simulink model "SimulationModel"  (R2014a)
settings: Solver=ode3  SolverMode=SingleTasking  StartTime=0.0  StopTime=180  FixedStep=deltaT  RelTol=1e-3
PostLoadFcn:
  | loadRobotParameters
  | 
  | allotedRunTime = 3*60; % [sec] Time allowed for run
  | 
  | % starting parameters
  | % The timer starts once the robot has moved a certain distance from the
  | % starting point
  | startPos = [50 50]; % [cm]
  | startingRadius = 10; % [cm]
  | 
  | % Target parameters
  | targetBoundaryRadius = 7; % [cm] radius considered at location
  | statTimeReq = 2.5; % [sec] minimum time robot must be at location
InitFcn:
  | close('all','force');
StartFcn:
  | reset(SimDisplay.getInstance());
undefined symbols (not defined in the file): AxleLength, deltaT, dT, EncL_init, EncR_init, EncRes, motorBiasLeft, motorBiasRight, motorDeadZoneFwd, motorDeadZoneRev, motorGainLeft, motorGainRight, TargetPositions, theta0, Ts, WheelRadius, x0, y0
libraries: simulink x5, opclib x1
CloseFcn:
  | close('all','force');
settings Model: PauseTimes=14  ExtModeTrigDuration=2  Creator=gpacitti  LastModifiedBy=arequet
settings DataIOCC: SignalLoggingSaveFormat=ModelDataLogs  SaveOutput=off  SignalLogging=off  DSMLogging=off  SaveTime=off
settings OptimizationCC: ExpressionDepthLimit=2147483647  OptimizeModelRefInitCode=on  LifeSpan=1
settings DebuggingCC: UnderspecifiedInitializationDetection=Classic  SolverPrmCheckMsg=none  MultiTaskDSMMsg=warning  MultiTaskCondExecSysMsg=none  ParameterPrecisionLossMsg=none  StateNameClashWarn=warning
settings HardwareCC: ProdLargestAtomicInteger=Long  ProdLargestAtomicFloat=Float  ProdEndianess=LittleEndian  ProdHWDeviceType=ARM Compatible->ARM 7
settings RTWCC: SystemTargetFile=ert.tlc  TemplateMakefile=ert_default_tmf  Description=Embedded Coder  RTWVerbose=off  ProcessScript=ert_make_rtw_hook  IncludeERTFirstTime=on
settings CodeAppCC: IgnoreCustomStorageClasses=off  CustomSymbolStrType=$N$R$M  InternalIdentifier=Classic
settings ERTTargetCC: ParMdlRefBuildCompliant=on  CompOptLevelCompliant=on  ConcurrentExecutionCompliant=on  ERTFirstTimeCompliant=on  ModelStepFunctionPrototypeControlCompliant=on  CPPClassGenCompliant=on  InlinedParameterPlacement=Hierarchical  ERTCustomFileTemplate=example_file_process.tlc
settings ConfigComp: Description=Design Verifier Custom Configuration Component  DVMaxTestCaseSteps=500  DVTestSuiteOptimization=CombinedObjectives (Nonlinear Extended)

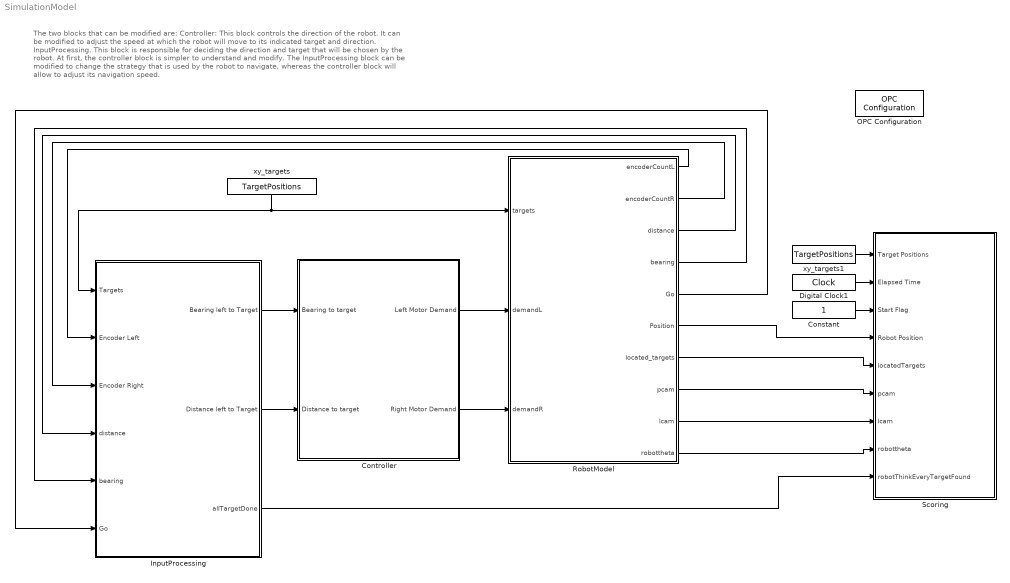
== system SimulationModel ==
  note: The two blocks that can be modified are:
      | Controller: This block controls the direction of the robot. It can be modified to adjust the speed at which the robot will move to its indicated target and direction.
      | InputProcessing. This block is responsible for deciding the direction and target that will be chosen by the robot.
      |
      | At first, the controller block is simpler to understand and modify.
      | The InputProcessing block can be modified to change the strategy that is used by the robot to navigate, whereas the controller block will allow to adjust its navigation speed.
  Constant : Constant  OutDataTypeStr=boolean
  Controller : Subsystem  TreatAsAtomicUnit=on
      mask Display: image('Arduino_Mega_2560.jpg',[0.75/2,0.3,0.25,0.4]);
  Digital Clock1 : DigitalClock  SampleTime=Ts
  InputProcessing : Subsystem
      mask Display: image('Arduino_Mega_2560.jpg',[0.75/2,0.3,0.25,0.3]);
  OPC Configuration : opclib/OPC Configuration  errMissingItems=Error  errReadWrite=Warn  errShutdown=Error  errRTViolation=None  rtEnable=on  speedup=1  showLatency=off  beingUsed=on
  RobotModel : Subsystem
      mask Display: image('robot_3d.jpg',[0.20,0.3,0.45,0.3]);
  Scoring : Subsystem
      mask Display: image('juge.jpg',[0.45,0.3,0.5,0.25]);
  xy_targets : Constant  Value=TargetPositions  OutDataTypeStr=single  SampleTime=1
  xy_targets1 : Constant  Value=TargetPositions  OutDataTypeStr=single  SampleTime=1
  wires:
  RobotModel/2(encoderCountR) -> InputProcessing/3(Encoder Right)
  RobotModel/1(encoderCountL) -> InputProcessing/2(Encoder Left)
  xy_targets/1 -> InputProcessing/1(Targets), RobotModel/1(targets)
  RobotModel/6(Position) -> Scoring/4(Robot Position)
  InputProcessing/2(Distance left to Target) -> Controller/2(Distance to target)
  InputProcessing/1(Bearing left to Target) -> Controller/1(Bearing to target)
  Controller/1(Left Motor Demand) -> RobotModel/2(demandL)
  Controller/2(Right Motor Demand) -> RobotModel/3(demandR)
  Constant/1 -> Scoring/3(Start Flag)
  Digital Clock1/1 -> Scoring/2(Elapsed Time)
  RobotModel/3(distance) -> InputProcessing/4(distance)
  RobotModel/4(bearing) -> InputProcessing/5(bearing)
  RobotModel/7(located_targets) -> Scoring/5(locatedTargets)
  RobotModel/8(pcam) -> Scoring/6(pcam)
  RobotModel/9(lcam) -> Scoring/7(lcam)
  RobotModel/10(robottheta) -> Scoring/8(robottheta)
  InputProcessing/3(allTargetDone) -> Scoring/9(robotThinkEveryTargetFound)
  xy_targets1/1 -> Scoring/1(Target Positions)
  RobotModel/5(Go) -> InputProcessing/6(Go)

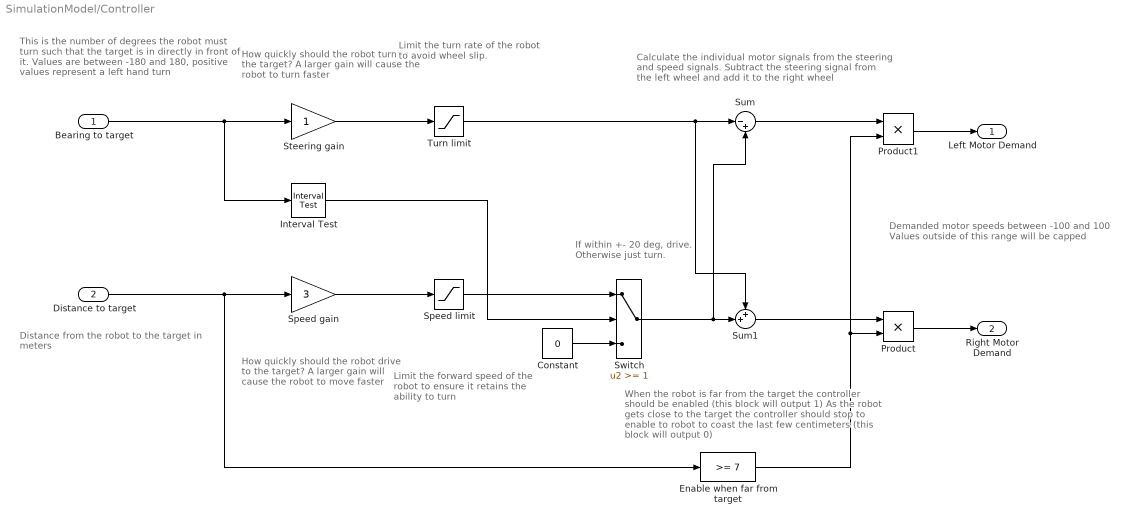
== system SimulationModel/Controller ==
  note: This is the number of degrees the robot
      | must turn such that the target is in directly
      | in front of it.
      | Values are between -180 and 180,
      | positive values represent a left hand turn
  note: Distance from the robot to the target
      | in meters
  note: Demanded motor speeds between -100 and 100
      | Values outside of this range will be capped
  note: How quickly should the robot turn
      | to the target? A larger gain will
      |  cause the robot to turn faster
  note: How quickly should the robot
      | drive to the target? A larger gain
      | will cause the robot to move
      | faster
  note: Limit the forward speed of the
      | robot to ensure it retains the
      | ability to turn
  note: When the robot is far from the target the controller
      | should be enabled (this block will output 1)
      | As the robot gets close to the target the controller
      | should stop to enable to robot to coast the last
      | few centimeters (this block will output 0)
  note: Calculate the individual motor signals from the
      | steering and speed signals. Subtract the steering
      | signal from the left wheel and add it to the right
      | wheel
  note: If within +- 20 deg, drive.
      | Otherwise just turn.
  note: Limit the turn rate of the
      | robot to avoid wheel slip.
  Bearing to target : Inport  OutDataTypeStr=single
  Distance to target : Inport  Port=2  PortDimensions=1  SampleTime=dT
  Constant : Constant  Value=0  OutDataTypeStr=single
  Enable when far from target : simulink/Logic and Bit Operations/Compare To Constant  relop=>=  const=7  OutDataTypeStr=uint8
  Interval Test : simulink/Logic and Bit Operations/Interval Test  IntervalClosedRight=on  uplimit=20  IntervalClosedLeft=on  lowlimit=-20  OutDataTypeStr=boolean
      settings: AttributesFormatString=|
      | Upper = %<uplimit>
      | Lower = %<lowlimit>
  Product : Product
  Product1 : Product
  Speed gain : Gain  Gain=3
  Speed limit : Saturate  UpperLimit=50  LowerLimit=0
      settings: AttributesFormatString=|
      | Upper = %<UpperLimit>
      | Lower = %<LowerLimit>
  Steering gain : Gain
  Sum : Sum  Inputs=|-+
  Sum1 : Sum  Inputs=++|
  Switch : Switch  Threshold=1
  Turn limit : Saturate  UpperLimit=50  LowerLimit=-50
      settings: AttributesFormatString=|
      | Upper = %<UpperLimit>
      | Lower = %<LowerLimit>
  Left Motor Demand : Outport  OutDataTypeStr=single
  Right Motor Demand : Outport  Port=2  OutDataTypeStr=single
  wires:
  Speed limit/1 -> Switch/1
  Turn limit/1 -> Sum1/1, Sum/1
  Constant/1 -> Switch/3
  Interval Test/1 -> Switch/2
  Sum/1 -> Product1/1
  Sum1/1 -> Product/1
  Bearing to target/1 -> Steering gain/1, Interval Test/1
  Switch/1 -> Sum1/2, Sum/2
  Enable when far from target/1 -> Product1/2, Product/2
  Product1/1 -> Left Motor Demand/1
  Product/1 -> Right Motor Demand/1
  Speed gain/1 -> Speed limit/1
  Steering gain/1 -> Turn limit/1
  Distance to target/1 -> Enable when far from target/1, Speed gain/1

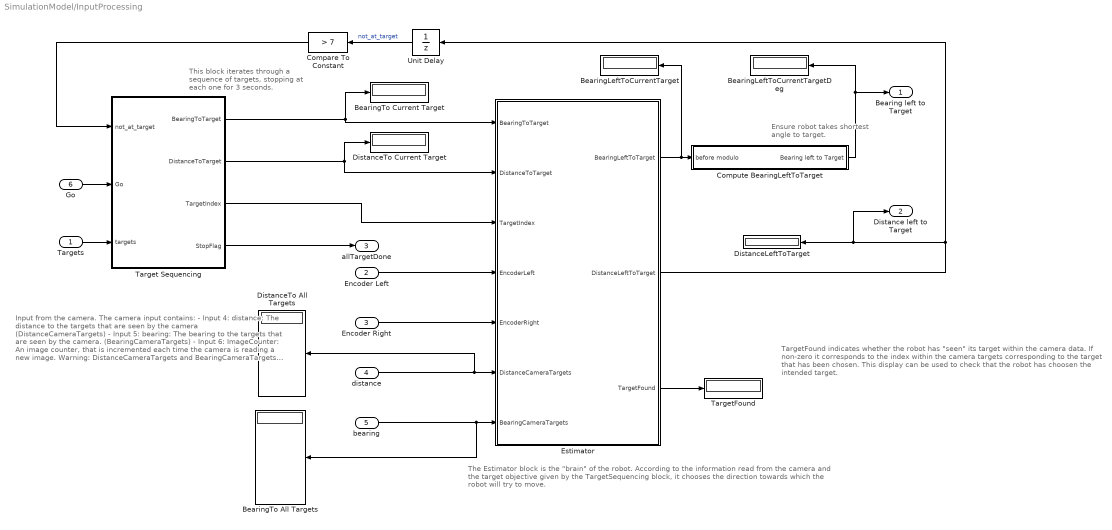
== system SimulationModel/InputProcessing ==
  note: TargetFound indicates whether the robot has "seen" its target within the camera
      | data.
      | If non-zero it corresponds to the index within the camera targets corresponding
      | to the target that has been chosen.
      |
      | This display can be used to check that the robot has choosen the intended
      | target.
  note: The Estimator block is the "brain" of the robot. According to the information read from the camera and the
      | target objective given by the TargetSequencing block, it chooses the direction towards which the robot
      | will try to move.
  note: Ensure robot takes shortest
      | angle to target.
  note: This block iterates through a
      | sequence of targets, stopping
      | at each one for 3 seconds.
  note: Input from the camera. The camera input contains:
      | - Input 4: distance: The distance to the targets that are seen by the
      |   camera (DistanceCameraTargets)
      | - Input 5: bearing: The bearing to the targets that are seen
      |   by the camera. (BearingCameraTargets)
      | - Input 6: ImageCounter: An image counter, that is incremented
      |   each time the camera is reading a new image.
      | Warning: DistanceCameraTargets and BearingCameraTargets
      | are the targets seen by the camera. So for instance, the
      | target 1 is the first target seen by the camera, but is not the
      | same target as the target at index 1 within the target sequencing
      | block.
  Targets : Inport
  Encoder Left : Inport  Port=2  OutDataTypeStr=class(intEncoder(0))
  Encoder Right : Inport  Port=3  OutDataTypeStr=class(intEncoder(0))
  distance : Inport  Port=4
  bearing : Inport  Port=5
  Go : Inport  Port=6
  BearingLeftToCurrentTarget : Display
  BearingLeftToCurrentTargetDeg : Display
  BearingTo All Targets : Display
  "BearingTo Current Target " : Display
  Compare To Constant : simulink/Logic and Bit Operations/Compare To Constant  relop=>  const=7  OutDataTypeStr=boolean
  Compute BearingLeftToTarget : Subsystem
  DistanceLeftToTarget : Display
  DistanceTo All Targets : Display
  DistanceTo Current Target : Display
  Estimator : MATLAB Function  TreatAsAtomicUnit=on
  Target Sequencing : Stateflow chart  TreatAsAtomicUnit=on
  TargetFound : Display
  Unit Delay : UnitDelay  SampleTime=dT
  Bearing left to Target : Outport  SampleTime=dT
  Distance left to Target : Outport  Port=2
  allTargetDone : Outport  Port=3
  wires:
  Go/1 -> Target Sequencing/2(Go)
  distance/1 -> DistanceTo All Targets/1, Estimator/6(DistanceCameraTargets)
  bearing/1 -> Estimator/7(BearingCameraTargets), BearingTo All Targets/1
  Target Sequencing/4(StopFlag) -> allTargetDone/1
  Compare To Constant/1 -> Target Sequencing/1(not_at_target)
  Compute BearingLeftToTarget/1(Bearing left to Target) -> BearingLeftToCurrentTargetDeg/1, Bearing left to Target/1
  Estimator/3(TargetFound) -> TargetFound/1
  Target Sequencing/3(TargetIndex) -> Estimator/3(TargetIndex)
  Estimator/2(DistanceLeftToTarget) -> DistanceLeftToTarget/1, Distance left to Target/1, Unit Delay/1
  Estimator/1(BearingLeftToTarget) -> BearingLeftToCurrentTarget/1, Compute BearingLeftToTarget/1(before modulo)
  Target Sequencing/1(BearingToTarget) -> Estimator/1(BearingToTarget), "BearingTo Current Target "/1
  Unit Delay/1 -> Compare To Constant/1  "not_at_target"
  Encoder Right/1 -> Estimator/5(EncoderRight)
  Target Sequencing/2(DistanceToTarget) -> Estimator/2(DistanceToTarget), DistanceTo Current Target/1
  Encoder Left/1 -> Estimator/4(EncoderLeft)
  Targets/1 -> Target Sequencing/3(targets)

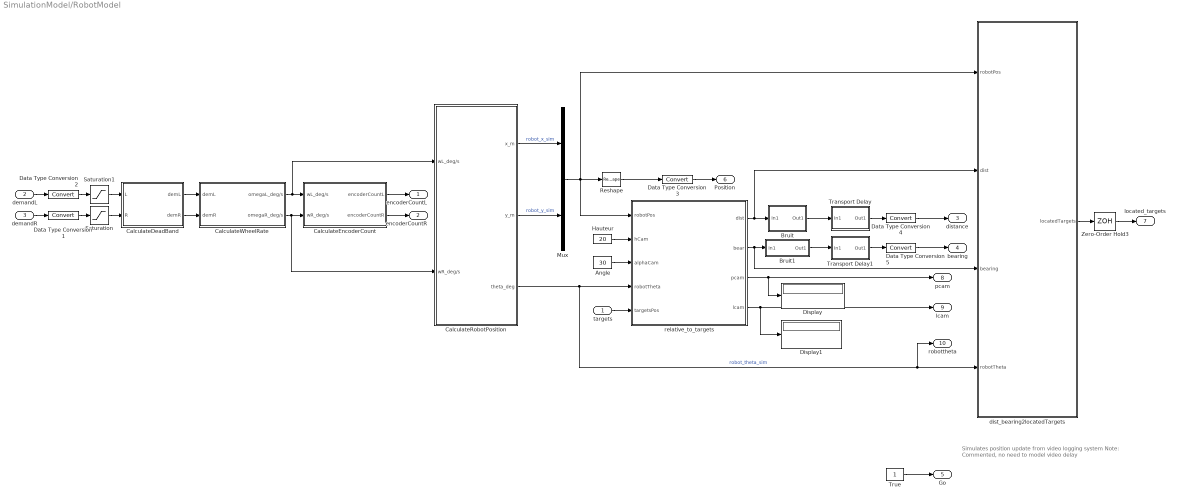
== system SimulationModel/RobotModel ==
  note: Simulates position update from video logging system
      | Note: Commented, no need to model video delay
  targets : Inport
  demandL : Inport  Port=2  SampleTime=0
  demandR : Inport  Port=3  SampleTime=0
  Angle : Constant  Value=30  OutMin=[30]  OutMax=[60]  SampleTime=0.2
  Bruit : Subsystem
  Bruit1 : Subsystem
  CalculateDeadBand : MATLAB Function  TreatAsAtomicUnit=on
  CalculateEncoderCount : Subsystem
  CalculateRobotPosition : Subsystem
  CalculateWheelRate : Subsystem
  Data Type Conversion{1..5} (5 alike) : DataTypeConversion
  Display : Display
  Display1 : Display
  Hauteur : Constant  Value=20  SampleTime=0.2
  Mux : Mux  Inputs=2
  Reshape : Reshape  OutputDimensionality=Row vector (2-D)
  Saturation : Saturate  UpperLimit=100  LowerLimit=-100
  Saturation1 : Saturate  UpperLimit=100  LowerLimit=-100
  Transport Delay : Subsystem  mask{timeDelay=0.250, initialOutput=zeros(size(6,1),1), initialBufferSize=1024, useFixedBufferSize=off, directFeedthoughOfInputDuringLinearization=off, padeOrder=0}
      mask prompts: initialOutput "Initial output"; initialBufferSize "Initial buffer size"; useFixedBufferSize "Use fixed buffer size"; directFeedthoughOfInputDuringLinearization "Direct feedthough of input during linearization"; padeOrder "Pade order (for linearization):"
  Transport Delay1 : Subsystem  mask{timeDelay=0.250, initialOutput=zeros(size(6,1),1), initialBufferSize=1024, useFixedBufferSize=off, directFeedthoughOfInputDuringLinearization=off, padeOrder=0}
      mask prompts: initialOutput "Initial output"; initialBufferSize "Initial buffer size"; useFixedBufferSize "Use fixed buffer size"; directFeedthoughOfInputDuringLinearization "Direct feedthough of input during linearization"; padeOrder "Pade order (for linearization):"
  True : Constant  OutMin=0  OutMax=1  SampleTime=0.1
  Zero-Order Hold3 : ZeroOrderHold  SampleTime=0.2
  dist_bearing2locatedTargets : MATLAB Function  TreatAsAtomicUnit=on
  relative_to_targets : MATLAB Function  TreatAsAtomicUnit=on
  encoderCountL : Outport  OutDataTypeStr=class(intEncoder(0))
  encoderCountR : Outport  Port=2  OutDataTypeStr=class(intEncoder(0))
  distance : Outport  Port=3  OutDataTypeStr=int16
  bearing : Outport  Port=4  OutDataTypeStr=int8
  Go : Outport  Port=5
  Position : Outport  Port=6
  located_targets : Outport  Port=7
  pcam : Outport  Port=8
  lcam : Outport  Port=9
  robottheta : Outport  Port=10
  wires:
  CalculateRobotPosition/1(x_m) -> Mux/1  "robot_x_sim"
  CalculateRobotPosition/2(y_m) -> Mux/2  "robot_y_sim"
  demandR/1 -> Data Type Conversion1/1
  demandL/1 -> Data Type Conversion2/1
  CalculateDeadBand/1(demL) -> CalculateWheelRate/1(demL)
  CalculateDeadBand/2(demR) -> CalculateWheelRate/2(demR)
  Saturation/1 -> CalculateDeadBand/2(R)
  Saturation1/1 -> CalculateDeadBand/1(L)
  CalculateEncoderCount/1(encoderCountL) -> encoderCountL/1
  CalculateEncoderCount/2(encoderCountR) -> encoderCountR/1
  CalculateRobotPosition/3(theta_deg) -> robottheta/1, dist_bearing2locatedTargets/4(robotTheta), relative_to_targets/4(robotTheta)  "robot_theta_sim"
  CalculateWheelRate/1(omegaL_deg/s) -> CalculateEncoderCount/1(wL_deg/s), CalculateRobotPosition/1(wL_deg/s)
  CalculateWheelRate/2(omegaR_deg/s) -> CalculateEncoderCount/2(wR_deg/s), CalculateRobotPosition/2(wR_deg/s)
  Data Type Conversion2/1 -> Saturation1/1
  Data Type Conversion1/1 -> Saturation/1
  Reshape/1 -> Data Type Conversion3/1
  Data Type Conversion3/1 -> Position/1
  targets/1 -> relative_to_targets/5(targetsPos)
  Zero-Order Hold3/1 -> located_targets/1
  dist_bearing2locatedTargets/1(locatedTargets) -> Zero-Order Hold3/1
  relative_to_targets/1(dist) -> Bruit/1(In1), dist_bearing2locatedTargets/2(dist)
  relative_to_targets/2(bear) -> Bruit1/1(In1), dist_bearing2locatedTargets/3(bearing)
  Transport Delay1/1(Out1) -> Data Type Conversion5/1
  Hauteur/1 -> relative_to_targets/2(hCam)
  Bruit1/1(Out1) -> Transport Delay1/1(In1)
  Angle/1 -> relative_to_targets/3(alphaCam)
  relative_to_targets/3(pcam) -> Display/1, pcam/1
  relative_to_targets/4(lcam) -> Display1/1, lcam/1
  Mux/1 -> dist_bearing2locatedTargets/1(robotPos), Reshape/1, relative_to_targets/1(robotPos)
  Bruit/1(Out1) -> Transport Delay/1(In1)
  Transport Delay/1(Out1) -> Data Type Conversion4/1
  Data Type Conversion4/1 -> distance/1
  Data Type Conversion5/1 -> bearing/1
  True/1 -> Go/1

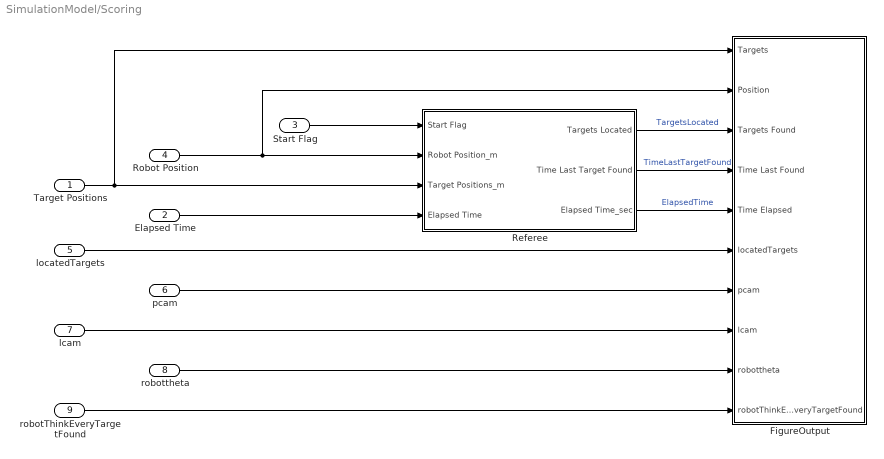
== system SimulationModel/Scoring ==
  Target Positions : Inport
  Elapsed Time : Inport  Port=2
  Start Flag : Inport  Port=3
  Robot Position : Inport  Port=4
  locatedTargets : Inport  Port=5
  pcam : Inport  Port=6
  lcam : Inport  Port=7
  robottheta : Inport  Port=8
  robotThinkEveryTargetFound : Inport  Port=9
  FigureOutput : Subsystem  TreatAsAtomicUnit=on  SimViewingDevice=on
  Referee : Subsystem
      mask Display: % image(imread('referee.png'))
  wires:
  Referee/1(Targets Located) -> FigureOutput/3(Targets Found)  "TargetsLocated"
  Referee/2(Time Last Target Found) -> FigureOutput/4(Time Last Found)  "TimeLastTargetFound"
  Referee/3(Elapsed Time_sec) -> FigureOutput/5(Time Elapsed)  "ElapsedTime"
  Start Flag/1 -> Referee/1(Start Flag)
  Robot Position/1 -> Referee/2(Robot Position_m), FigureOutput/2(Position)
  Elapsed Time/1 -> Referee/4(Elapsed Time)
  Target Positions/1 -> FigureOutput/1(Targets), Referee/3(Target Positions_m)
  locatedTargets/1 -> FigureOutput/6(locatedTargets)
  pcam/1 -> FigureOutput/7(pcam)
  lcam/1 -> FigureOutput/8(lcam)
  robottheta/1 -> FigureOutput/9(robottheta)
  robotThinkEveryTargetFound/1 -> FigureOutput/10(robotThinkEveryTargetFound)

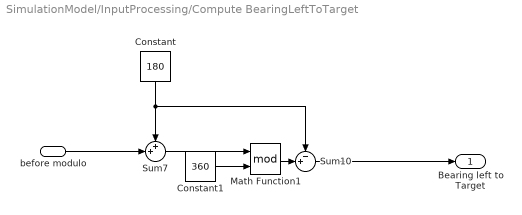
== system SimulationModel/InputProcessing/Compute BearingLeftToTarget ==
  before modulo : Inport
  Constant : Constant  Value=180  OutDataTypeStr=Inherit: Inherit via back propagation
  Constant1 : Constant  Value=360  OutDataTypeStr=Inherit: Inherit via back propagation
  Math Function1 : Math  Operator=mod  SaturateOnIntegerOverflow=on
  Sum10 : Sum  Inputs=-+|
  Sum7 : Sum  Inputs=++|
  Bearing left to Target : Outport  SampleTime=dT
  wires:
  before modulo/1 -> Sum7/2
  Sum10/1 -> Bearing left to Target/1
  Math Function1/1 -> Sum10/2
  Constant1/1 -> Math Function1/2
  Sum7/1 -> Math Function1/1
  Constant/1 -> Sum10/1, Sum7/1

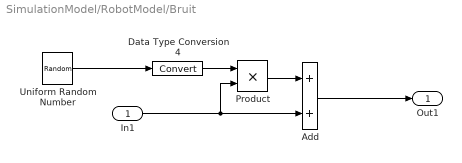
== system SimulationModel/RobotModel/Bruit ==
  In1 : Inport
  Add : Sum
  Data Type Conversion4 : DataTypeConversion
  Product : Product
  Uniform Random Number : UniformRandomNumber  Minimum=-0.05  Maximum=0.05  SampleTime=0.2
  Out1 : Outport
  wires:
  In1/1 -> Add/2, Product/2
  Product/1 -> Add/1
  Uniform Random Number/1 -> Data Type Conversion4/1
  Data Type Conversion4/1 -> Product/1
  Add/1 -> Out1/1

== system SimulationModel/RobotModel/Bruit1 ==
  In1 : Inport
  Add : Sum
  Data Type Conversion4 : DataTypeConversion
  Product : Product
  Uniform Random Number : UniformRandomNumber  Minimum=-0.05  Maximum=0.05  SampleTime=0.2
  Out1 : Outport
  wires:
  Data Type Conversion4/1 -> Product/1
  Uniform Random Number/1 -> Data Type Conversion4/1
  Product/1 -> Add/1
  In1/1 -> Add/2, Product/2
  Add/1 -> Out1/1

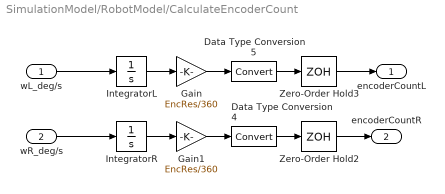
== system SimulationModel/RobotModel/CalculateEncoderCount ==
  wL_deg/s : Inport
  wR_deg/s : Inport  Port=2
  Data Type Conversion4 : DataTypeConversion
  Data Type Conversion5 : DataTypeConversion
  Gain : Gain  Gain=EncRes/360
  Gain1 : Gain  Gain=EncRes/360
  IntegratorL : Integrator  InitialCondition=EncL_init
  IntegratorR : Integrator  InitialCondition=EncR_init
  Zero-Order Hold2 : ZeroOrderHold  SampleTime=0.1
  Zero-Order Hold3 : ZeroOrderHold  SampleTime=0.1
  encoderCountL : Outport
  encoderCountR : Outport  Port=2
  wires:
  Data Type Conversion5/1 -> Zero-Order Hold3/1
  Data Type Conversion4/1 -> Zero-Order Hold2/1
  wR_deg/s/1 -> IntegratorR/1
  wL_deg/s/1 -> IntegratorL/1
  IntegratorL/1 -> Gain/1
  IntegratorR/1 -> Gain1/1
  Zero-Order Hold2/1 -> encoderCountR/1
  Zero-Order Hold3/1 -> encoderCountL/1
  Gain/1 -> Data Type Conversion5/1
  Gain1/1 -> Data Type Conversion4/1

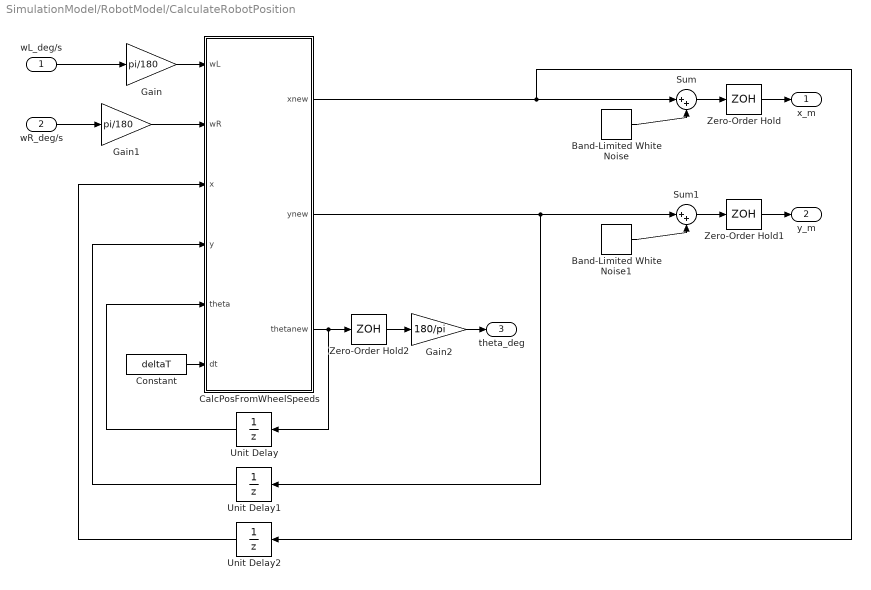
== system SimulationModel/RobotModel/CalculateRobotPosition ==
  wL_deg/s : Inport
  wR_deg/s : Inport  Port=2
  Band-Limited White Noise : simulink/Sources/Band-Limited White Noise  Cov=1e-5  Ts=dT  seed=[23341]
  Band-Limited White Noise1 : simulink/Sources/Band-Limited White Noise  Cov=1e-5  Ts=dT  seed=[23342]
  CalcPosFromWheelSpeeds : MATLAB Function  TreatAsAtomicUnit=on
  Constant : Constant  Value=deltaT
  Gain : Gain  Gain=pi/180
  Gain1 : Gain  Gain=pi/180
  Gain2 : Gain  Gain=180/pi
  Sum : Sum  Inputs=|++
  Sum1 : Sum  Inputs=|++
  Unit Delay : UnitDelay  InitialCondition=theta0  SampleTime=-1
  Unit Delay1 : UnitDelay  InitialCondition=y0  SampleTime=-1
  Unit Delay2 : UnitDelay  InitialCondition=x0  SampleTime=-1
  Zero-Order Hold : ZeroOrderHold  SampleTime=Ts
  Zero-Order Hold1 : ZeroOrderHold  SampleTime=Ts
  Zero-Order Hold2 : ZeroOrderHold  SampleTime=Ts
  x_m : Outport
  y_m : Outport  Port=2
  theta_deg : Outport  Port=3
  wires:
  Constant/1 -> CalcPosFromWheelSpeeds/6(dt)
  Unit Delay/1 -> CalcPosFromWheelSpeeds/5(theta)
  CalcPosFromWheelSpeeds/2(ynew) -> Sum1/1, Unit Delay1/1
  Unit Delay1/1 -> CalcPosFromWheelSpeeds/4(y)
  CalcPosFromWheelSpeeds/1(xnew) -> Unit Delay2/1, Sum/1
  Unit Delay2/1 -> CalcPosFromWheelSpeeds/3(x)
  Band-Limited White Noise/1 -> Sum/2
  Band-Limited White Noise1/1 -> Sum1/2
  Sum/1 -> Zero-Order Hold/1
  Sum1/1 -> Zero-Order Hold1/1
  CalcPosFromWheelSpeeds/3(thetanew) -> Zero-Order Hold2/1, Unit Delay/1
  wL_deg/s/1 -> Gain/1
  wR_deg/s/1 -> Gain1/1
  Zero-Order Hold2/1 -> Gain2/1
  Zero-Order Hold1/1 -> y_m/1
  Zero-Order Hold/1 -> x_m/1
  Gain/1 -> CalcPosFromWheelSpeeds/1(wL)
  Gain1/1 -> CalcPosFromWheelSpeeds/2(wR)
  Gain2/1 -> theta_deg/1

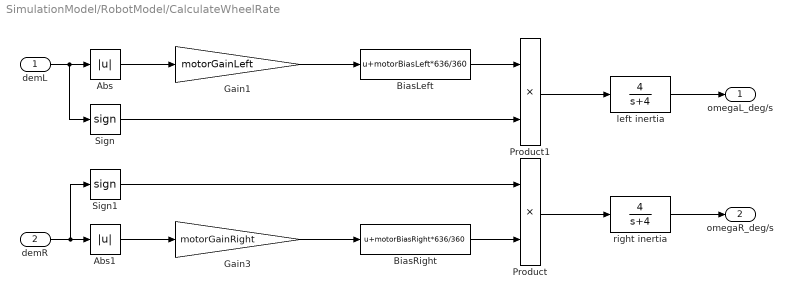
== system SimulationModel/RobotModel/CalculateWheelRate ==
  demL : Inport
  demR : Inport  Port=2
  " left inertia" : TransferFcn  Numerator=[4]  Denominator=[1 4]
  Abs : Abs
  Abs1 : Abs
  BiasLeft : Bias  Bias=motorBiasLeft*636/360
  BiasRight : Bias  Bias=motorBiasRight*636/360
  Gain1 : Gain  Gain=motorGainLeft
  Gain3 : Gain  Gain=motorGainRight
  Product : Product  RndMeth=Zero
  Product1 : Product  RndMeth=Zero
  Sign : Signum
  Sign1 : Signum
  right inertia : TransferFcn  Numerator=[4]  Denominator=[1 4]
  omegaL_deg/s : Outport
  omegaR_deg/s : Outport  Port=2
  wires:
  Gain3/1 -> BiasRight/1
  Abs1/1 -> Gain3/1
  demR/1 -> Sign1/1, Abs1/1
  Abs/1 -> Gain1/1
  demL/1 -> Sign/1, Abs/1
  BiasRight/1 -> Product/2
  BiasLeft/1 -> Product1/1
  Product/1 -> right inertia/1
  Sign/1 -> Product1/2
  Sign1/1 -> Product/1
  Product1/1 -> " left inertia"/1
  Gain1/1 -> BiasLeft/1
  " left inertia"/1 -> omegaL_deg/s/1
  right inertia/1 -> omegaR_deg/s/1

== system SimulationModel/RobotModel/Transport Delay ==
  In1 : Inport
  Data Type Conversion : DataTypeConversion  OutDataTypeStr=double
  Data Type Conversion4 : DataTypeConversion  OutDataTypeStr=single
  Transport Delay : TransportDelay  DelayTime=timeDelay  InitialOutput=initialOutput  BufferSize=initialBufferSize  PadeOrder=padeOrder
  Zero-Order Hold : ZeroOrderHold  SampleTime=Ts
  Out1 : Outport
  wires:
  Transport Delay/1 -> Data Type Conversion4/1
  Data Type Conversion/1 -> Transport Delay/1
  Data Type Conversion4/1 -> Zero-Order Hold/1
  In1/1 -> Data Type Conversion/1
  Zero-Order Hold/1 -> Out1/1

== system SimulationModel/RobotModel/Transport Delay1 ==
  In1 : Inport
  Data Type Conversion : DataTypeConversion  OutDataTypeStr=double
  Data Type Conversion4 : DataTypeConversion  OutDataTypeStr=single
  Transport Delay : TransportDelay  DelayTime=timeDelay  InitialOutput=initialOutput  BufferSize=initialBufferSize  PadeOrder=padeOrder
  Zero-Order Hold : ZeroOrderHold  SampleTime=Ts
  Out1 : Outport
  wires:
  In1/1 -> Data Type Conversion/1
  Data Type Conversion4/1 -> Zero-Order Hold/1
  Data Type Conversion/1 -> Transport Delay/1
  Transport Delay/1 -> Data Type Conversion4/1
  Zero-Order Hold/1 -> Out1/1

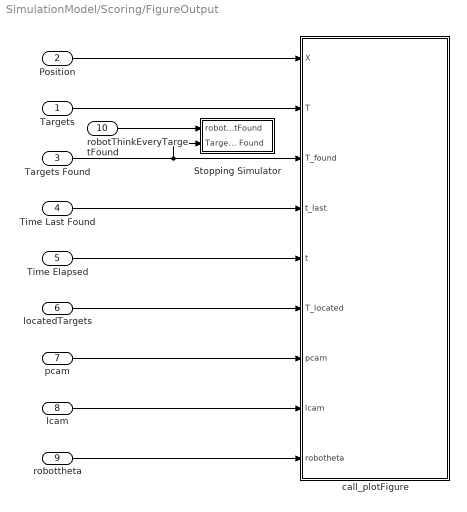
== system SimulationModel/Scoring/FigureOutput ==
  Targets : Inport
  Position : Inport  Port=2
  Targets Found : Inport  Port=3
  Time Last Found : Inport  Port=4
  Time Elapsed : Inport  Port=5
  locatedTargets : Inport  Port=6
  pcam : Inport  Port=7
  lcam : Inport  Port=8
  robottheta : Inport  Port=9
  robotThinkEveryTargetFound : Inport  Port=10
  Stopping Simulator : Subsystem
  call_plotFigure : MATLAB Function  TreatAsAtomicUnit=on
  wires:
  Position/1 -> call_plotFigure/1(X)
  Targets/1 -> call_plotFigure/2(T)
  Targets Found/1 -> call_plotFigure/3(T_found), Stopping Simulator/2(Targets Found)
  Time Last Found/1 -> call_plotFigure/4(t_last)
  Time Elapsed/1 -> call_plotFigure/5(t)
  locatedTargets/1 -> call_plotFigure/6(T_located)
  pcam/1 -> call_plotFigure/7(pcam)
  lcam/1 -> call_plotFigure/8(lcam)
  robottheta/1 -> call_plotFigure/9(robotheta)
  robotThinkEveryTargetFound/1 -> Stopping Simulator/1(robotThinkEveryTargetFound)

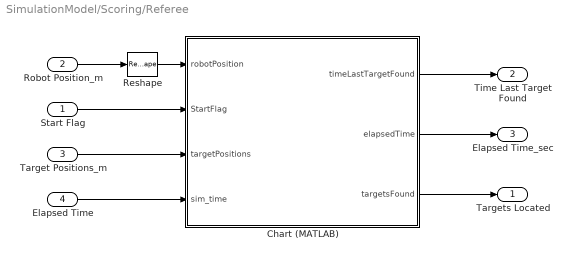
== system SimulationModel/Scoring/Referee ==
  Start Flag : Inport  OutDataTypeStr=boolean  SampleTime=Ts
  Robot Position_m : Inport  Port=2  SampleTime=Ts
  Target Positions_m : Inport  Port=3  SampleTime=Ts
  Elapsed Time : Inport  Port=4  SampleTime=Ts
  Chart (MATLAB) : Stateflow chart  TreatAsAtomicUnit=on
  Reshape : Reshape  OutputDimensionality=Row vector (2-D)
  Targets Located : Outport
  Time Last Target Found : Outport  Port=2  PortDimensions=1
  Elapsed Time_sec : Outport  Port=3  PortDimensions=1
  wires:
  Chart (MATLAB)/1(timeLastTargetFound) -> Time Last Target Found/1
  Chart (MATLAB)/3(targetsFound) -> Targets Located/1
  Robot Position_m/1 -> Reshape/1
  Start Flag/1 -> Chart (MATLAB)/2(StartFlag)
  Reshape/1 -> Chart (MATLAB)/1(robotPosition)
  Target Positions_m/1 -> Chart (MATLAB)/3(targetPositions)
  Chart (MATLAB)/2(elapsedTime) -> Elapsed Time_sec/1
  Elapsed Time/1 -> Chart (MATLAB)/4(sim_time)

== system SimulationModel/Scoring/FigureOutput/Stopping Simulator ==
  robotThinkEveryTargetFound : Inport
  Targets Found : Inport  Port=2
  Data Type Conversion : DataTypeConversion  OutDataTypeStr=double
  Logical Operator : Logic  Operator=OR  AllPortsSameDT=off  OutDataTypeStr=boolean
  MinMax : MinMax
  Stop Simulation : Stop
  wires:
  Targets Found/1 -> Data Type Conversion/1
  Data Type Conversion/1 -> MinMax/1
  Logical Operator/1 -> Stop Simulation/1
  robotThinkEveryTargetFound/1 -> Logical Operator/1
  MinMax/1 -> Logical Operator/2

== matlab function SimulationModel/InputProcessing/Estimator ==
  data: BearingToTarget input; DistanceToTarget input; TargetIndex input; BearingLeftToTarget output; EncoderLeft input; DistanceLeftToTarget output; EncoderRight input; DistanceCameraTargets input; BearingCameraTargets input; TargetFound output; AxleLength parameter; WheelRadius parameter; EncRes parameter
function [BearingLeftToTarget, DistanceLeftToTarget, TargetFound] = ...
    estimator(BearingToTarget, DistanceToTarget, TargetIndex, EncoderLeft, ...
    EncoderRight, DistanceCameraTargets, BearingCameraTargets,...
    AxleLength, WheelRadius, EncRes)
%#codegen
%% This function computes the direction of the robot using:
% - The target that is selected by the target sequencer (i.e. the target
%   that the robot is intending to reach):
%   + BearingToTarget, DistanceToTarget, TargetIndex
% - The information from the wheel encoders:
%   + EncoderLeft (left wheel)
%   + EncoderRight (right wheel)
% - The information sent by the camera:
%   + DistanceCameraTargets: an array storing the distance to the camera
%     for each of the targets that are seen by the camera.
%   + BearingCameraTargets: an array storing the orientation to the 
%     target for each of the targets that are seen by the camera.
%   + ImageCounter: The acquisition counter from the camera: as the 
%     camera frequency is lower than the frequency of this block, this
%     block may be executed several time with the same information from
%     the camera.
%     ImageCounter can be used to indicate that the information is "fresh".


%% Index of the current target that the robot will try to reach.
% Storing it persistently allows us to determine when a new 
% target is selected
persistent  cur_target_index 

%% Values of the encoders left and right when reaching the
% last target.
persistent encoder_left_prev_target encoder_right_prev_target 

%% Those two variables are storing the position of the target 
% relative to the robot's position.
% They are updated when the robot is moving.
persistent distance_to_target bearing_to_target 
%% Stores the last image counter received from the camera. 
% It is used to check whether a new image has been received from the
% camera, since this block is executed more frequently than the camera.

if isempty(cur_target_index)
    %% Initializes the persistent values to default values
    cur_target_index = uint8(0);
    encoder_left_prev_target = int32(0);
    encoder_right_prev_target = int32(0);
    distance_to_target = single(0);
    bearing_to_target = single(0);
end

%% In the case where the target has changed, updates the target information.
if (cur_target_index ~= TargetIndex)
    cur_target_index = TargetIndex;
    % Save encoders value
    encoder_left_prev_target = EncoderLeft;
    encoder_right_prev_target = EncoderRight;
    bearing_to_target = BearingToTarget;
    distance_to_target = DistanceToTarget;
end

%%%%%%%%%%%%%%%%%%%%%
% Robot distance and angle based on encoders
% Axle length = 160mm
% Wheel diameter = 66.5mm
% Encoder = 12*53 = 636 ticks per wheel turn

%% Updates the position information from the encoders information.
dL = single(EncoderLeft - encoder_left_prev_target) * 2 * WheelRadius * pi / EncRes;
dR = single(EncoderRight - encoder_right_prev_target) * 2 * WheelRadius * pi / EncRes;
CurrentDistance = ((dL + dR)/2);
DistanceLeftToTarget = distance_to_target - CurrentDistance;

% Angle from prev target
CurrentBearing = single(((dR - dL)*180) / (AxleLength*pi));

BearingLeftToTarget = bearing_to_target - CurrentBearing;
% Ensure our robot angle stays within a single revolution
%BearingLeftToTarget = single(mod(BearingLeftToTarget,360));


%% Correction using the camera.
%
% In the case where a new image is received from the camera, 
% try to adjust the direction.
% This adjustment is only performed if the robot has traveled
% at least 5cm since the last target. This delay is here to 
% prevent changing the direction too often because of the
% camera input delay.
TargetFound=uint8(0);
dist_left = int16(DistanceLeftToTarget);
if(CurrentDistance > 5 && dist_left> 20 )
    %% Search for the target within the targets that are seen by the 
    % camera.
    % A target is chosen if it is at less than 10cms of the searched 
    % target, and within 36 degree.
    % In the case where several candidate targets are seen, the target
    % chosen is the target that is the closest to the expected distance.
    for ind=1:length(DistanceCameraTargets)
        if(DistanceCameraTargets(ind) > 5 )
            if(abs(DistanceCameraTargets(ind) - dist_left)<10 && ...
                    abs(BearingCameraTargets(ind))<36 )
                if (TargetFound==0 || abs(DistanceCameraTargets(TargetFound) - ...
                        dist_left)>abs(DistanceCameraTargets(ind) - dist_left))
                    TargetFound=uint8(ind);
                end
            end
        end
    end

    if ( TargetFound ~= 0)
        %% In the case where a target has been found, adjust the 
        % information.
        DistanceLeftToTarget = single(DistanceCameraTargets(TargetFound));   % data from camera
        BearingLeftToTarget = single(BearingCameraTargets(TargetFound))/2;   % data from camera
        % Reset encoders
        encoder_left_prev_target = EncoderLeft;
        encoder_right_prev_target = EncoderRight;
        bearing_to_target = BearingLeftToTarget;
        distance_to_target = DistanceLeftToTarget;
    else
        %% Not target found.
        % TODO: This code could be removed (TargetFound is already 0), but
        TargetFound=uint8(0);
        DistanceLeftToTarget=DistanceLeftToTarget;  %#ok<ASGSL> data from encoders
        BearingLeftToTarget=BearingLeftToTarget;    %#ok<ASGSL> data from encoders
    end
end

== matlab function SimulationModel/RobotModel/CalculateDeadBand ==
  data: L input; demL output; R input; demR output; motorDeadZoneFwd parameter; motorDeadZoneRev parameter
function [demL, demR] = deadband(L, R, motorDeadZoneFwd, motorDeadZoneRev)
%#codegen

if R < motorDeadZoneRev
    demR = R;
elseif R > motorDeadZoneFwd
    demR = R;
else
    demR = 0;
end

if L < motorDeadZoneRev
    demL = L;
elseif L > motorDeadZoneFwd
    demL = L;
else
    demL = 0;
end

== stateflow chart SimulationModel/InputProcessing/Target Sequencing ==
  settings: description=The index of the current target that the robot will try to reach.
  state This block is chosing target that the robot will try to reach. [group]
    It returns the direction and distance to the next target from the
    previous target (i.e. the direction and distance are not adjustedwhen the robot is moving).
    Its inputs are:
    - not_at_target: indicates whether the robot is on a target or not.
    - targets: the list of targets, in the order that they will be
    reached.
    Its outputs are:
    - BearingToTarget: The bearing to the next target, from the previous
    target.
    - DistanceToTarget: The distance to the next target, from the previous
    target.
    - TargetIndex: the index of the target.
    - StopFlag: set to true when the robot has moved through all the targets.
  state MovingToTarget
  state Wait
    entry:
    wait_timer = pause_time;
    during:
    wait_timer = wait_timer - 0.1;
  state Finished
    entry:
    StopFlag = 1;
  (default) -> (junction 34) : { TargetIndex = uint8(0); prev_bearing = single(0); prev_target = single([50;50]); }
  (junction 34) -> MovingToTarget : % Advance to the first target
      | { nextTarget(); }
  Wait -> MovingToTarget [order 2] : % Finished waiting. Advance to the next target.
      | [ wait_timer <= 0 && TargetIndex < length(targets) ]
      | { nextTarget(); }
  MovingToTarget -> MovingToTarget [order 1] : [ ~Go ]
  MovingToTarget -> Wait [order 2] : % Target reached
      | [   ~not_at_target ]
  Wait -> Finished [order 1] : % No more targets
      | [ wait_timer <= 0 && TargetIndex >= length(targets) ]
  data: pause_time constant single =3.0; not_at_target input; Go input; targets input; BearingToTarget output =0; DistanceToTarget output =0; TargetIndex output uint8 =0; StopFlag output =0; prev_target local single size=2 =single([50;50]); prev_bearing local =single(0); wait_timer local
  data pause_time settings: description=The time in seconds the robot will wait when it reaches a target before selecting the new target.
  data not_at_target settings: description=Indicates whether the robot is supposed to be on a target or not.
  data targets settings: description=The list of targets that the robot will try to reach, in the order that they will be reached.
  data BearingToTarget settings: description=The bearing to the next target, from the previous target.
  data DistanceToTarget settings: description=The distance to the next target, from the previous target.
  data TargetIndex settings: description=The index of the current target.
  data StopFlag settings: description=Set to true when the robot has moved through all the targets.
  data prev_target settings: description=The position of the previous target.
  data prev_bearing settings: description=The previous bearing to the target.
  data wait_timer settings: description=Timer that is used to wait 'pause_time' when positioned on a target.
  function nextTarget:
    | function nextTarget
    | %% This function advance to the next target, and updates the outputs
    | % DistanceToTarget, BearingToTarget and TargetIndex accordingly
    | TargetIndex = TargetIndex + 1;
    | current_target_pos = [targets(TargetIndex,1);targets(TargetIndex,2)];
    | 
    | % Distance from previous target to current target.
    | DistanceToTarget = (norm(current_target_pos-prev_target));
    | 
    | % Compute bearing between the two target positions.
    | dy = current_target_pos(2)-prev_target(2);
    | dx = current_target_pos(1)-prev_target(1);
    | BearingToTarget = (atan2d(dy,dx));
    | % Adjust the bearing with the previous bearing
    | BearingToTarget = BearingToTarget-prev_bearing;
    | 
    | % Update the "previous" values
    | prev_target=[targets(TargetIndex,1);targets(TargetIndex,2)];
    | prev_bearing=prev_bearing+BearingToTarget;

== stateflow chart SimulationModel/Scoring/Referee/Chart (MATLAB) ==
  state Standby
    entry:
    numTargets = size(targetPositions,1);
    targetsFound = false(size(targetPositions,1),1);
    timeLastTargetFound = 0;
    elapsedTime = 0;
    numTargetsFound = 0;
  state Running
    entry: startTiming;
    during:
    elapsedTime = getTiming;
    [nearLocation, currentTarget] = testIfNearLocation(robotPosition, targetPositions, targetBoundaryRadius);
    state NearLocation
      entry: snapshotTime = elapsedTime;
    state Roaming
    Roaming -> NearLocation : [nearLocation == true]
    (default) -> Roaming
    NearLocation -> Roaming [order 2] : [nearLocation == false]
    NearLocation -> (junction 43) [order 1] : [(elapsedTime - snapshotTime) > statTimeReq]
    (junction 44) -> Roaming
    (junction 43) -> (junction 44) : {[targetsFound, timeLastTargetFound] = ...
        | updateTargetsFound(targetsFound, currentTarget, timeLastTargetFound,elapsedTime);
        | numTargetsFound = sum(targetsFound);}
  state Finished
  Finished -> Standby : [StartFlag == false]
  (default) -> Standby
  Standby -> Running : [StartFlag == true &&...
      | distancefrom(robotPosition, startPos) < startingRadius ]
  Running -> Standby [order 2] : [StartFlag == false]
  Running -> Finished [order 1] : [numTargetsFound == numTargets ||...
      |  elapsedTime >= allotedRunTime-sqrt(eps)]
  data: et function_output; tfound_in function_input; currentT function_input; tfound_out function_output; lastTime_in function_input; lastTime_out function_output; time function_input; robotPos function_input; targetPos function_input; proximityVal function_input; nearLoc function_output; currentLoc function_output; pos function_input; x0 function_input; d function_output; startPos parameter; allotedRunTime parameter; statTimeReq parameter; startingRadius parameter; robotPosition input; targetBoundaryRadius parameter; StartFlag input; targetPositions input; timeLastTargetFound output; nearLocation local; numTargetsFound local; elapsedTime output; numTargets local; currentTarget local; targetsFound output; snapshotTime local; local_t local; sim_time input
  function startTiming:
    | function startTiming
    | global local_t sim_time
    | 
    | if strcmp(coder.target,'rtw')
    |     coder.ceval('tic',int32(2));
    | else
    |     local_t = sim_time;
    | end
  function et = getTiming:
    | function et = getTiming
    | global sim_time local_t
    | 
    | lt = 0;
    | 
    | if strcmp(coder.target,'rtw')
    |     coder.ceval('toc',coder.wref(lt),int32(2));
    | else
    |     lt = sim_time - local_t;
    | end
    | 
    | et = lt;
  function [tfound_out, lastTime_out] = updateTargetsFound(tfound_in, currentT, lastTime_in, time):
    | function [tfound_out, lastTime_out] = updateTargetsFound(tfound_in, currentT, lastTime_in, time)
    | 
    | if any(tfound_in & currentT) %is this an existing target
    |     lastTime_out = lastTime_in;
    | else
    |     lastTime_out = time;
    | end
    | 
    | tfound_out = tfound_in | currentT; %update list of found targets
  function [nearLoc, currentLoc] = testIfNearLocation(robotPos, targetPos, proximityVal):
    | function [nearLoc, currentLoc] = testIfNearLocation(robotPos, targetPos, proximityVal)
    | %#codegen
    | delta = bsxfun(@minus, targetPos, robotPos);
    | dist = sum(delta.^2,2);
    | 
    | currentLoc = dist <= proximityVal^2;
    | nearLoc = any(currentLoc);
  function d = distancefrom(pos,x0):
    | function d = distancefrom(pos,x0)
    | d = sqrt(sum((pos-x0).^2));

== matlab function SimulationModel/Scoring/FigureOutput/call_plotFigure ==
  data: X input; T input; T_found input; t_last input; t input; T_located input; pcam input; lcam input; robotheta input
function fcn(X, T, T_found, t_last, t, T_located,pcam,lcam,robotheta)
coder.extrinsic('plotFigure');

plotFigure(X, T, T_found, t_last, t, T_located,pcam,lcam,robotheta);

== matlab function SimulationModel/RobotModel/relative_to_targets ==
  data: robotPos input size=[1 2]; hCam input; alphaCam input; robotTheta input size=1; dist output; bear output; targetsPos input; pcam output; lcam output
function [dist,bear, pcam ,lcam] = targets(robotPos,hCam,alphaCam,robotTheta,targetsPos)
%#codegen
%% TARGETS Returns distance and bearing for each target relative to robot
%
% Distances and positions are in cm
% Angles are in degrees
%
% Inputs
%   - hCam: Cam height (from ground)
%   - targetsPos: Position of targets (X,Y)
%   - robotPos: Robot position (X,Y)
%   - robotTheta: Robot angle
%
% Outputs
%   - dist (array nx1 with n=nb targets): Distances for each target, 
%       if a target cannot be seen by the camera associated distance 
%       is equal to -1
%   - bearing (array nx1 with n=nb targets): Angles for each target, 
%       if a target cannot be seen by the camera associated angle is 
%       equal to -1
%

% Get camera field of vision
% [pcam,lcam]=camera(hCam);
% betaCam = 21 ;
% etaCam = 27 ;
% [pcam, lcam] = cameraAnalytic(hCam,90-alphaCam, betaCam, etaCam);
pcam = [25, 105];
lcam = [27, 108];

% Convert target position to robot reference
[x,y] = world2robot(robotPos(1),robotPos(2),robotTheta,targetsPos(:,1),targetsPos(:,2));

% Get distance and bearing for each point relative to robot
[distance,bearing] = isincamera(pcam,lcam,x,y);

% sort by descending order and return 6 elements
[distance,idxsort] = sort(distance,'descend');
bearing = bearing(idxsort);
if length(distance)<6
    dist = [distance;zeros(6-length(distance),1)];
    bear = [bearing;zeros(6-length(bearing),1)] ;
else
    dist = distance(1:6);
    bear = bearing(1:6);
end


function [p_cam,l_cam]=camera(h_camera)
%% CAMERA Returns camera field of vision
%
% Input
%   - h_camera: Camera height (in cm)
%
% Outputs
%   - p_cam: Camera vision depth, 2 values: minimal and maximal depth for 
%       the camera position. Depth corresponds to Y axis. Unit = cm.
%   - l_cam: Camera vision width, 2 values: minimal and maximal width for 
%       the camera position. Width corresponds to X axis. Unit = cm.
%

% Calibration values
% ------------------
% Height
height=[10 23 41 52];
% Depth
pmin=[13 34 40 50];
pmax=[100 160 240 300];
% Width
lmin=[20 50 62 62];
lmax=[110 205 300 360];

% Polynomial approximation with 1rst degree polynom (y = a*x+b)
coef_pmin=polyfit(height(2:end),pmin(2:end),1);
coef_pmax=polyfit(height(2:end),pmax(2:end),1);
coef_lmin=polyfit(height(2:end),lmin(2:end),1);
coef_lmax=polyfit(height(2:end),lmax(2:end),1);

% Depth and width are calculated with polynomial approximation
p_cam=[ polyval(coef_pmin,h_camera) polyval(coef_pmax,h_camera)];
l_cam=[ polyval(coef_lmin,h_camera) polyval(coef_lmax,h_camera)];


function [p_cam, l_cam] = cameraAnalytic(h_camera, alpha_camera, beta_camera, eta_camera)
%
%
% Inputs
%   - h_camera      : Camera height (in cm)
%   - alpha_camera  : angle between the vertical (z-axis) and the camera 
%   - beta_camera   : vertical angle of view of camera / 2 (in degrees)
%   - eta_camera    : horizontal angle of view of camera / 2 (in degrees)
%
% Outputs
%   - p_cam: Camera vision depth, 2 values: minimal and maximal depth for 
%       the camera position. Depth corresponds to Y axis. Unit = cm.
%   - l_cam: Camera vision width, 2 values: minimal and maximal width for 
%       the camera position. Width corresponds to X axis. Unit = cm.
%

l_cam = zeros(1,2);
p_cam = zeros(1,2);
d1 = h_camera * tand( alpha_camera + beta_camera ) ;
d2 = h_camera * tand( alpha_camera - beta_camera ) ;
k1 = h_camera / cosd( alpha_camera - beta_camera ) ;
k2 = h_camera / cosd( alpha_camera + beta_camera ) ;
f1 = k1 * tand( eta_camera ) ;
f2 = k2 * tand( eta_camera ) ;

l_cam(1) = 2 * f1 ;
l_cam(2) = 2 * f2 ;
p_cam(1) = d2 ;
p_cam(2) = d1 ;
p_far_factor = -7;
p_close_factor = 2;
p_cam(2) = p_cam(2) + p_far_factor;
p_cam(1) = p_cam(1) + p_close_factor;



function [x_new,y_new]=world2robot(x_robot,y_robot,theta_robot,x_world,y_world)
% WORLD2ROBOT Convert coordinates from world to robot
%
% Inputs
%   - x_robot: Robot X position (in world reference)
%   - y_robot: Robot Y position (in world reference)
%   - theta_robot: Robot angle  (in world reference)
%   - x_world: X value(s) to convert (in world reference)
%   - y_world: Y value(s) to convert (in world reference)
%
% Outpus
%   - x_new: Point(s) coordinate (X) in robot reference
%   - y_new: Point(s) coordinate (Y) in robot reference

% Translate coordinates reference
x_dif=x_world-x_robot;
y_dif=y_world-y_robot;

% Rotate coordinates reference
% x_new=x_dif*cosd(theta_robot)-y_dif*sind(theta_robot);
% y_new=x_dif*sind(theta_robot)+y_dif*cosd(theta_robot);
x_new = cosd(theta_robot)*x_dif + sind(theta_robot)*y_dif;
y_new = cosd(theta_robot)*y_dif - sind(theta_robot)*x_dif;
% see http://www.mathematics-online.org/inhalt/aussage/aussage444/

% TODO We have identified that the sign of converted coordinates is the
% opposite of the expected but we don't have an explanation for that
% x_new = -x_new;
% y_new = -y_new;

function [dist,bearing]=isincamera(p,l,x,y)
%% ISINCAMERA Distance and angle from current robot position
%
% Inputs
%   - p (2 elements vector): Minimal and maximal depth for camera (Y axis)
%   - l (2 elements vector): Minimal and maximal width for camera (X axis)
%   - x (vector): X coordinate of point(s)
%   - y (vector): Y coordinate of point(s)
%
% Outputs
%   - dist (vector): Distance of each point from camera (robot), -1 if
%       point cannot be seen by camera.
%   - bearing (vector): Angle of each point from camera (robot), -1 if
%       point cannot be seen by camera.
%

% Calculate coefficients for lines that defines the camera field of vision
% Field vision limits in Y axis are constants (y = p(1) or y = p(2))
c1=polyfit(p(1:2),[-l(1)/2 -l(2)/2],1);
c2=polyfit(p(1:2),[l(1)/2 l(2)/2],1);

% To be visible a point must match all the following criterion
%   - Y >= minimal depth
%   - Y <= maximal depth
%   - X >= - (width for current Y) / 2
%   - X <=   (width for current Y) / 2
%

%isvisible = y>=p(1) & y<=p(2) & (x>=polyval(c1,y) & x<=polyval(c2,y));
isvisible = x>=p(1) & x<=p(2) & (y>=polyval(c1,x) & y<=polyval(c2,x));

% Calculate distance and bearing for all points
dist = sqrt(x.^2 + y.^2);
% bearing = atan2d(y,x);
bearing = atan2d(x,-y)-90;

% Replace values by -1 for points that are not visible
dist(~isvisible) = 0;
bearing(~isvisible) = 0;

== matlab function SimulationModel/RobotModel/dist_bearing2locatedTargets ==
  data: robotPos input; dist input; locatedTargets output; bearing input; robotTheta input
function locatedTargets = fcn(robotPos, dist, bearing, robotTheta)
%#codegen

loc = dist>0;

locatedTargetsX = zeros(size(dist));
locatedTargetsY = locatedTargetsX;

targetTheta = robotTheta+bearing(loc);

locatedTargetsX(loc) = robotPos(1)+dist(loc).*cosd(targetTheta);
locatedTargetsY(loc) = robotPos(2)+dist(loc).*sind(targetTheta);

locatedTargets = [locatedTargetsX, locatedTargetsY];

== matlab function SimulationModel/RobotModel/CalculateRobotPosition/CalcPosFromWheelSpeeds ==
  data: wL input; wR input; x input; y input; theta input; dt input; xnew output; ynew output; thetanew output; AxleLength parameter; WheelRadius parameter
function [xnew,ynew, thetanew] = calcRobPos(wL, wR, x, y, theta, dt, AxleLength, WheelRadius)
%#codegen

vL = wL*WheelRadius;
vR = wR*WheelRadius;

if(vL == vR)
    xdot = vL * cos(theta);
    ydot = vR * sin(theta); 
    xnew = x + xdot*dt;
    ynew = y + ydot*dt;
    thetanew = theta;
else
    R = (AxleLength/2)*(vL + vR)/(vR - vL);
    omega = (vR - vL)/AxleLength;
    
    ICCx = x - R*sin(theta);
    ICCy = y + R*cos(theta);
    rotMat = [cos(omega*dt) -sin(omega*dt) 0;...
              sin(omega*dt) cos(omega*dt) 0;...
              0 0 1];
    newpos = rotMat*[x - ICCx; y-ICCy; theta] + [ICCx;ICCy;omega*dt];
    xnew = newpos(1);
    ynew = newpos(2);
    thetanew = newpos(3);
end

if thetanew > 2*pi
    thetanew = thetanew - (2*pi);
elseif thetanew < 0
    thetanew = thetanew + (2*pi);
end

end
